simulink model "test_pkt_fifo_10_1"  (Simulink 7.0)
settings: Solver=ode45  StartTime=0.0  StopTime=2000  RelTol=1e-3
libraries: xbsIndex_r4 x102, xps_library x7, xbsReplacements_r4 x4, casper_library x3
settings Model: Creator=Jason Manley  LastModifiedBy=dsp
settings DebuggingCC: SaveWithParameterizedLinksMsg=none  SignalResolutionControl=TryResolveAllWithWarning  MultiTaskDSMMsg=warning  MultiTaskCondExecSysMsg=none  StrictBusMsg=None
settings RTWCC: IncludeERTFirstTime=on
settings GRTTargetCC: TargetFcnLib=ansi_tfl_tmw.mat

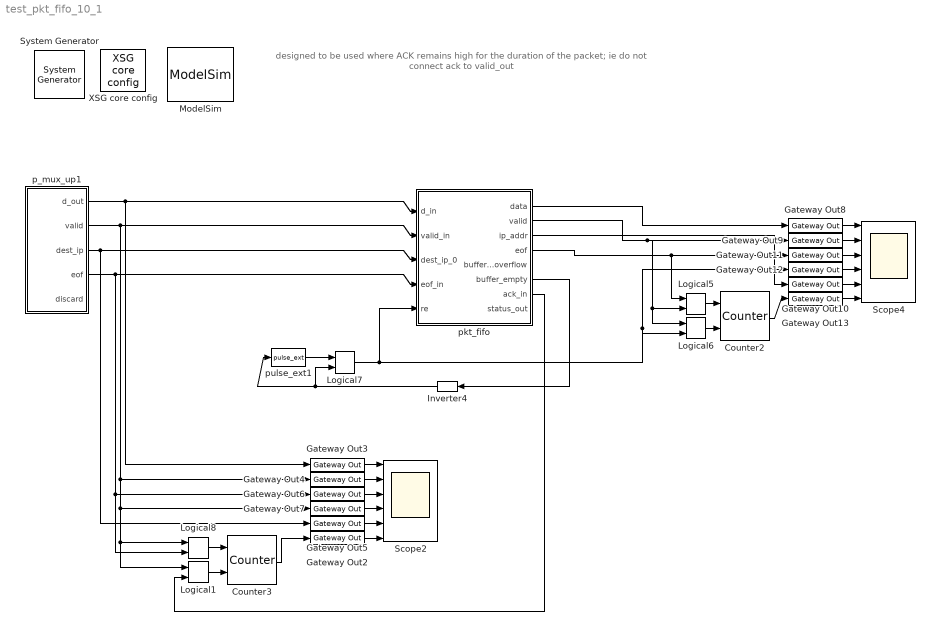
== system test_pkt_fifo_10_1 ==
  note: designed to be used where ACK remains high for the duration of the packet;
      | ie do not connect ack to valid_out
  " System Generator" : xbsIndex_r4/ System Generator  Tag=genX  SystemSampleTime=-1  xilinxfamily=Virtex2P  part=xc2vp70  speed=-7  package=ff1704  synthesis_tool=XST  clock_wrapper=Clock Enables  directory=./test_10gbe_mux_pack/sysgen  testbench=off  simulink_period=1  sysclk_period=4.878  dcm_input_clock_period=100  incr_netlist=off  trim_vbits=Everywhere in SubSystem  dbl_ovrd=According to Block Masks  core_generation=According to Block Masks  run_coregen=off  deprecated_control=off  eval_field=0  block_type=sysgen
      settings: block_version=10.1.3
  Counter2 : xbsIndex_r4/Counter  cnt_type=Free Running  cnt_to=Inf  operation=Up  start_count=0  cnt_by_val=1  arith_type=Unsigned  n_bits=8  bin_pt=0  load_pin=off  rst=on  en=on  explicit_period=off  period=1  dbl_ovrd=off  use_behavioral_HDL=off  use_rpm=on  implementation=Fabric  block_type=counter
      settings: xl_area=[0, 0, 0, 0, 0, 0, 0]
  Counter3 : xbsIndex_r4/Counter  cnt_type=Free Running  cnt_to=Inf  operation=Up  start_count=0  cnt_by_val=1  arith_type=Unsigned  n_bits=8  bin_pt=0  load_pin=off  rst=on  en=on  explicit_period=off  period=1  dbl_ovrd=off  use_behavioral_HDL=off  use_rpm=on  implementation=Fabric  block_type=counter
      settings: xl_area=[0, 0, 0, 0, 0, 0, 0]
  Gateway Out{2..13} (12 alike) : xbsIndex_r4/Gateway Out  hdl_port=on  timing_constraint=None  locs_specified=off  LOCs={}  block_type=gatewayout
      settings: infoedit="Gateway out block.  Converts Xilinx fixed point inputs into ouputs of type Simulink integer, double, or fixed point.<P><P>Hardware notes:  In hardware these blocks become top level output ports or are discarded, depending on how they are configured."  xl_area=[0, 0, 0, 0, 0, 0, 0]  block_version=10.1.3
  Inverter4 : xbsIndex_r4/Inverter  Orientation=left  en=off  latency=0  dbl_ovrd=off  block_type=inv
      settings: xl_area=[0, 0, 0, 0, 0, 0, 0]
  Logical{1,5..6,8} (4 alike) : xbsIndex_r4/Logical  logical_function=AND  inputs=2  en=off  latency=0  precision=Full  arith_type=Unsigned  n_bits=8  bin_pt=2  align_bp=on  dbl_ovrd=off  block_type=logical
      settings: xl_area=[0, 0, 0, 0, 0, 0, 0]
  Logical7 : xbsIndex_r4/Logical  logical_function=OR  inputs=2  en=off  latency=0  precision=Full  arith_type=Unsigned  n_bits=8  bin_pt=2  align_bp=on  dbl_ovrd=off  block_type=logical
      settings: xl_area=[0, 0, 0, 0, 0, 0, 0]
  ModelSim : xbsIndex_r4/ModelSim  dir=./modelsim  waveform=on  leave_open=on  skip_compile=off  use_unisim=off  custom_scripts=off  startup_timeout=40  block_type=hdlcosim
      settings: infoedit="Allow other blocks to schedule HDL co-simulation tasks.<P><P>Note that selecting \"Skip compilation\" when inappropriate can cause simulation errors and failures. Please refer to the block help for details."  block_version=10.1.3
  Scope2 : Scope  NumInputPorts=6
      settings: YMin=410.4~-1~-1~-1~0~-5  YMax=453.6~1~1~1~1~5  SaveName=ScopeData5
  Scope4 : Scope  NumInputPorts=6
      settings: YMin=410.4~-1~-1~-1~0~-5  YMax=453.6~1~1~1~1~5  SaveName=ScopeData7
  XSG core config : xps_library/XSG core config  Tag=xps:xsg  SystemSampleTime=-1  hw_sys=BEE2_usr  ibob_linux=off  clk_src=sys_clk  iBOB_clk_src=sys_clk  BEE2_ctrl_clk_src=sys_clk  BEE2_usr_clk_src=sys_clk  ROACH_clk_src=arb_clk  CORR_clk_src=sys_clk  gpio_clk_io_group=iBOB:sma  gpio_clk_bit_index=0  clk_rate=100  sample_period=1  synthesis_tool=XST  mpc_type=powerpc405
  p_mux_up1 : Subsystem
  pkt_fifo : Subsystem
      settings: AttributesFormatString=|
      | Max 1024 data words.
      | Max 32 pkts.
  pulse_ext1 : casper_library/Misc/pulse_ext  SystemSampleTime=-1  pulse_len=10
  wires:
  Gateway Out8/1 -> Scope4/1
  Gateway Out9/1 -> Scope4/2
  Gateway Out11/1 -> Scope4/3
  Gateway Out12/1 -> Scope4/4
  Gateway Out10/1 -> Scope4/5
  Gateway Out13/1 -> Scope4/6
  Gateway Out3/1 -> Scope2/1
  Gateway Out4/1 -> Scope2/2
  Gateway Out6/1 -> Scope2/3
  Gateway Out7/1 -> Scope2/4
  Gateway Out5/1 -> Scope2/5
  p_mux_up1/1(d_out) -> Gateway Out3/1, pkt_fifo/1(d_in)
  p_mux_up1/2(valid) -> Gateway Out4/1, Gateway Out7/1, Logical8/1, Logical1/1, pkt_fifo/2(valid_in)
  p_mux_up1/3(dest_ip) -> Gateway Out5/1, pkt_fifo/3(dest_ip_0)
  p_mux_up1/4(eof) -> Gateway Out6/1, Logical8/2, pkt_fifo/4(eof_in)
  pkt_fifo/1(data) -> Gateway Out8/1
  pkt_fifo/2(valid) -> Gateway Out9/1, Logical5/2, Logical6/1
  Logical5/1 -> Counter2/1
  Counter2/1 -> Gateway Out13/1
  pkt_fifo/4(eof) -> Logical5/1, Gateway Out11/1
  Logical7/1 -> Gateway Out12/1, Logical6/2, pkt_fifo/5(re)
  pkt_fifo/3(ip_addr) -> Gateway Out10/1
  Logical6/1 -> Counter2/2
  pulse_ext1/1 -> Logical7/1
  Logical8/1 -> Counter3/1
  Logical1/1 -> Counter3/2
  Gateway Out2/1 -> Scope2/6
  Counter3/1 -> Gateway Out2/1
  pkt_fifo/7(ack_in) -> Logical1/2
  pkt_fifo/6(buffer_empty) -> Inverter4/1
  Inverter4/1 -> pulse_ext1/1, Logical7/2

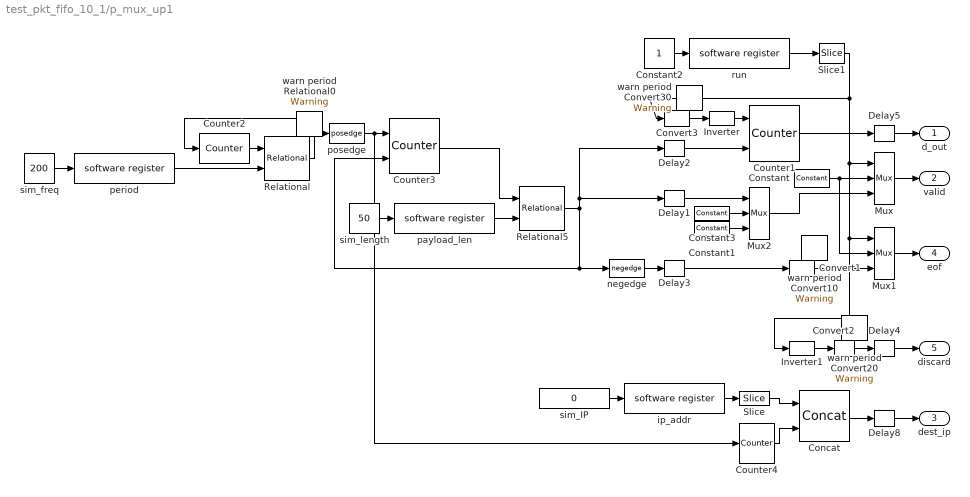
== system test_pkt_fifo_10_1/p_mux_up1 ==
  Concat : xbsIndex_r4/Concat  num_inputs=2  dbl_ovrd=off  block_type=concat
      settings: block_version=10.1.3
  Constant : xbsIndex_r4/Constant  arith_type=Boolean  const=0  n_bits=1  bin_pt=0  explicit_period=on  period=1  equ=P=C  opselect=C  inp2=PCIN>>17  opr=+  inp1=P  carry=CIN  dbl_ovrd=off  block_type=constant
  Constant1 : xbsIndex_r4/Constant  arith_type=Boolean  const=1  n_bits=1  bin_pt=0  explicit_period=off  period=1  equ=P=C  opselect=C  inp2=PCIN>>17  opr=+  inp1=P  carry=CIN  dbl_ovrd=off  block_type=constant
  Constant2 : Constant  OutDataType=sfix(16)  OutScaling=2^0
  Constant3 : xbsIndex_r4/Constant  arith_type=Boolean  const=0  n_bits=1  bin_pt=0  explicit_period=off  period=1  equ=P=C  opselect=C  inp2=PCIN>>17  opr=+  inp1=P  carry=CIN  dbl_ovrd=off  block_type=constant
  Convert1 : xbsIndex_r4/Convert  arith_type=Boolean  n_bits=8  bin_pt=6  quantization=Truncate  overflow=Wrap  latency=0  dbl_ovrd=off  pipeline=off  block_type=convert
      settings: xl_area=[0, 0, 0, 0, 0, 0, 0]  block_version=10.1.3
  Convert2 : xbsIndex_r4/Convert  arith_type=Boolean  n_bits=8  bin_pt=6  quantization=Truncate  overflow=Wrap  latency=0  dbl_ovrd=off  pipeline=off  block_type=convert
      settings: xl_area=[0, 0, 0, 0, 0, 0, 0]  block_version=10.1.3
  Convert3 : xbsIndex_r4/Convert  arith_type=Boolean  n_bits=8  bin_pt=6  quantization=Truncate  overflow=Wrap  latency=0  dbl_ovrd=off  pipeline=off  block_type=convert
      settings: xl_area=[0, 0, 0, 0, 0, 0, 0]  block_version=10.1.3
  Counter1 : xbsIndex_r4/Counter  cnt_type=Free Running  cnt_to=Inf  operation=Up  start_count=0  cnt_by_val=1  arith_type=Unsigned  n_bits=64  bin_pt=0  load_pin=off  rst=on  en=on  explicit_period=off  period=1  dbl_ovrd=off  use_behavioral_HDL=off  use_rpm=off  implementation=Fabric  block_type=counter
      settings: xl_area=[0, 0, 0, 0, 0, 0, 0]
  Counter2 : xbsIndex_r4/Counter  cnt_type=Free Running  cnt_to=Inf  operation=Up  start_count=1  cnt_by_val=1  arith_type=Unsigned  n_bits=32  bin_pt=0  load_pin=off  rst=on  en=off  explicit_period=on  period=1  dbl_ovrd=off  use_behavioral_HDL=off  use_rpm=on  implementation=Fabric  block_type=counter
      settings: xl_area=[0, 0, 0, 0, 0, 0, 0]
  Counter3 : xbsIndex_r4/Counter  cnt_type=Free Running  cnt_to=1023  operation=Up  start_count=0  cnt_by_val=1  arith_type=Unsigned  n_bits=32  bin_pt=0  load_pin=off  rst=on  en=on  explicit_period=on  period=1  dbl_ovrd=off  use_behavioral_HDL=off  use_rpm=on  implementation=Fabric  block_type=counter
      settings: xl_area=[0, 0, 0, 0, 0, 0, 0]
  Counter4 : xbsIndex_r4/Counter  cnt_type=Free Running  cnt_to=1023  operation=Up  start_count=0  cnt_by_val=1  arith_type=Unsigned  n_bits=2  bin_pt=0  load_pin=off  rst=off  en=on  explicit_period=on  period=1  dbl_ovrd=off  use_behavioral_HDL=off  use_rpm=on  implementation=Fabric  block_type=counter
      settings: xl_area=[0, 0, 0, 0, 0, 0, 0]
  Delay{1..5} (5 alike) : xbsIndex_r4/Delay  en=off  latency=1  dbl_ovrd=off  reg_retiming=on  block_type=delay
      settings: xl_area=[0, 0, 0, 0, 0, 0, 0]
  Delay8 : xbsIndex_r4/Delay  en=off  latency=2  dbl_ovrd=off  reg_retiming=on  block_type=delay
      settings: xl_area=[0, 0, 0, 0, 0, 0, 0]
  Inverter : xbsIndex_r4/Inverter  en=off  latency=0  dbl_ovrd=off  block_type=inv
      settings: xl_area=[0, 0, 0, 0, 0, 0, 0]
  Inverter1 : xbsIndex_r4/Inverter  en=off  latency=0  dbl_ovrd=off  block_type=inv
      settings: xl_area=[0, 0, 0, 0, 0, 0, 0]
  Mux : xbsIndex_r4/Mux  inputs=2  en=off  latency=1  precision=Full  arith_type="Signed  (2's comp)"  n_bits=8  bin_pt=2  quantization=Truncate  overflow=Wrap  dbl_ovrd=off  block_type=mux
      settings: xl_area=[0, 0, 0, 0, 0, 0, 0]
  Mux1 : xbsIndex_r4/Mux  inputs=2  en=off  latency=1  precision=Full  arith_type="Signed  (2's comp)"  n_bits=8  bin_pt=2  quantization=Truncate  overflow=Wrap  dbl_ovrd=off  block_type=mux
      settings: xl_area=[0, 0, 0, 0, 0, 0, 0]
  Mux2 : xbsIndex_r4/Mux  inputs=2  en=off  latency=1  precision=Full  arith_type="Signed  (2's comp)"  n_bits=8  bin_pt=2  quantization=Truncate  overflow=Wrap  dbl_ovrd=off  block_type=mux
      settings: xl_area=[0, 0, 0, 0, 0, 0, 0]
  Relational : xbsIndex_r4/Relational  mode=a>=b  en=off  latency=0  dbl_ovrd=off  block_type=relational
      settings: xl_area=[0, 0, 0, 0, 0, 0, 0]  block_version=10.1.3
  Relational5 : xbsIndex_r4/Relational  mode=a<b  en=off  latency=0  dbl_ovrd=off  block_type=relational
      settings: xl_area=[0, 0, 0, 0, 0, 0, 0]  block_version=10.1.3
  Slice : xbsIndex_r4/Slice  nbits=30  boolean_output=off  mode=Upper Bit Location + Width  bit1=0  base1=MSB of Input  bit0=0  base0=LSB of Input  dbl_ovrd=off  block_type=slice
      settings: infoedit="Extracts a given range of bits from each input sample and presents it at the output.  The output type is ordinarily unsigned with binary point at zero, but can be Boolean when the slice is one bit wide.<P><P>Hardware notes: In hardware this block costs nothing."  block_version=10.1.3
  Slice1 : xbsIndex_r4/Slice  nbits=1  boolean_output=off  mode=Lower Bit Location + Width  bit1=1  base1=MSB of Input  bit0=0  base0=LSB of Input  dbl_ovrd=off  block_type=slice
      settings: infoedit="Extracts a given range of bits from each input sample and presents it at the output.  The output type is ordinarily unsigned with binary point at zero, but can be Boolean when the slice is one bit wide.<P><P>Hardware notes: In hardware this block costs nothing."  block_version=10.1.3
  ip_addr : xps_library/software register  Tag=xps:sw_reg  SystemSampleTime=-1  io_dir=From Processor  arith_type=Unsigned  bitwidth=32  bin_pt=0  sample_period=1  gw_name=test_pkt_fifo_10_1_p_mux_up1_ip_addr_user_data_out
      link override test_pkt_buffer_10_1_p_mux_up1_ip_addr_user_data_out: arith_type=Unsigned  n_bits=32  bin_pt=0  period=1
      link override test_pkt_fifo_10_1_p_mux_up1_ip_addr_user_data_out: arith_type=Unsigned  n_bits=32  bin_pt=0  period=1
  negedge : casper_library/Misc/negedge  Tag=Rising Edge Detector  SystemSampleTime=-1
  payload_len : xps_library/software register  Tag=xps:sw_reg  SystemSampleTime=-1  io_dir=From Processor  arith_type=Unsigned  bitwidth=32  bin_pt=0  sample_period=1  gw_name=test_pkt_fifo_10_1_p_mux_up1_payload_len_user_data_out
      link override test_pkt_buffer_10_1_p_mux_up1_payload_len_user_data_out: arith_type=Unsigned  n_bits=32  bin_pt=0  period=1
      link override test_pkt_fifo_10_1_p_mux_up1_payload_len_user_data_out: arith_type=Unsigned  n_bits=32  bin_pt=0  period=1
  period : xps_library/software register  Tag=xps:sw_reg  SystemSampleTime=-1  io_dir=From Processor  arith_type=Unsigned  bitwidth=32  bin_pt=0  sample_period=1  gw_name=test_pkt_fifo_10_1_p_mux_up1_period_user_data_out
      link override test_pkt_buffer_10_1_p_mux_up1_period_user_data_out: arith_type=Unsigned  n_bits=32  bin_pt=0  period=1
      link override test_pkt_fifo_10_1_p_mux_up1_period_user_data_out: arith_type=Unsigned  n_bits=32  bin_pt=0  period=1
  posedge : casper_library/Misc/pulse_ext/posedge  Tag=Rising Edge Detector  SystemSampleTime=-1
  run : xps_library/software register  Tag=xps:sw_reg  SystemSampleTime=-1  io_dir=From Processor  arith_type=Unsigned  bitwidth=32  bin_pt=0  sample_period=1  gw_name=test_pkt_fifo_10_1_p_mux_up1_run_user_data_out
      link override test_pkt_buffer_10_1_p_mux_up1_run_user_data_out: arith_type=Unsigned  n_bits=32  bin_pt=0  period=1
      link override test_pkt_fifo_10_1_p_mux_up1_run_user_data_out: arith_type=Unsigned  n_bits=32  bin_pt=0  period=1
  sim_IP : Constant  Value=0  OutDataType=sfix(16)  OutScaling=2^0
  sim_freq : Constant  Value=200  OutDataType=sfix(16)  OutScaling=2^0
  sim_length : Constant  Value=50  OutDataType=sfix(16)  OutScaling=2^0
  warn period Convert10 : xbsReplacements_r4/Warning  SystemSampleTime=-1  period=1
  warn period Convert20 : xbsReplacements_r4/Warning  SystemSampleTime=-1  period=1
  warn period Convert30 : xbsReplacements_r4/Warning  SystemSampleTime=-1  period=1
  warn period Relational0 : xbsReplacements_r4/Warning  SystemSampleTime=-1  period=1
  d_out : Outport  OutDataType=sfix(16)  OutScaling=2^0
  valid : Outport  Port=2  OutDataType=sfix(16)  OutScaling=2^0
  dest_ip : Outport  Port=3  OutDataType=sfix(16)  OutScaling=2^0
  eof : Outport  Port=4  OutDataType=sfix(16)  OutScaling=2^0
  discard : Outport  Port=5  OutDataType=sfix(16)  OutScaling=2^0
  wires:
  Counter2/1 -> Relational/1
  Relational/1 -> posedge/1, Counter2/1
  Counter1/1 -> Delay5/1
  negedge/1 -> Delay3/1
  period/1 -> Relational/2
  sim_freq/1 -> period/1
  sim_IP/1 -> ip_addr/1
  Relational5/1 -> Counter3/2, negedge/1, Delay2/1, Delay1/1
  Counter3/1 -> Relational5/1
  posedge/1 -> Counter3/1, Counter4/1
  sim_length/1 -> payload_len/1
  payload_len/1 -> Relational5/2
  Mux/1 -> valid/1
  Constant/1 -> Mux/2, Mux1/2
  Mux1/1 -> eof/1
  Delay3/1 -> Convert1/1
  Convert1/1 -> Mux1/3
  Delay5/1 -> d_out/1
  Delay8/1 -> dest_ip/1
  run/1 -> Slice1/1
  Constant2/1 -> run/1
  Slice1/1 -> Mux/1, Mux1/1, Inverter1/1, Convert3/1
  Delay4/1 -> discard/1
  Mux2/1 -> Mux/3
  Inverter/1 -> Counter1/1
  Delay2/1 -> Counter1/2
  Convert3/1 -> Inverter/1
  Constant3/1 -> Mux2/2
  Constant1/1 -> Mux2/3
  Inverter1/1 -> Convert2/1
  Delay1/1 -> Mux2/1
  Convert2/1 -> Delay4/1
  ip_addr/1 -> Slice/1
  Counter4/1 -> Concat/2
  Slice/1 -> Concat/1
  Concat/1 -> Delay8/1

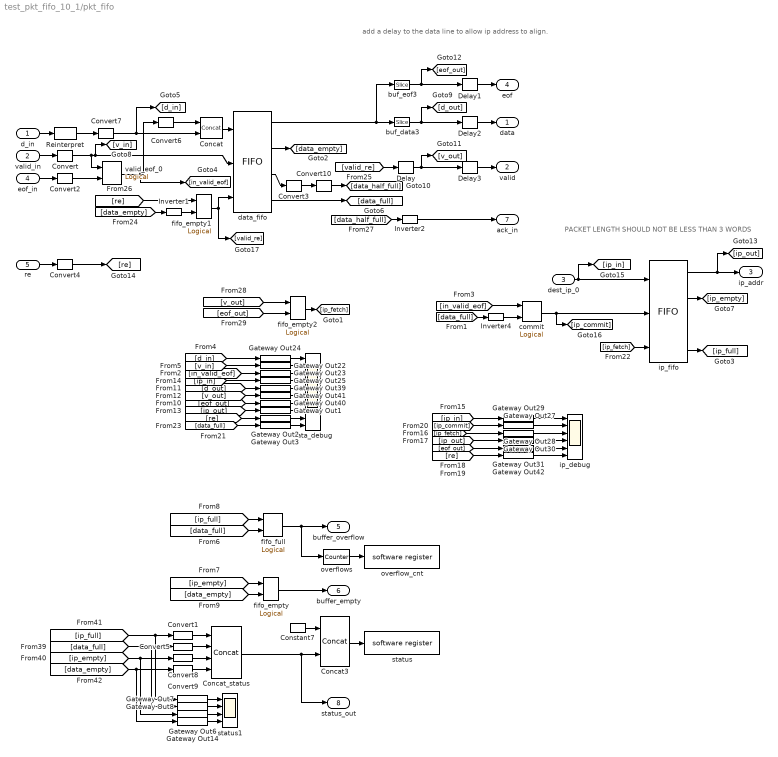
== system test_pkt_fifo_10_1/pkt_fifo ==
  note: PACKET LENGTH SHOULD NOT BE LESS THAN 3 WORDS
  note: add a delay to the data line to allow
      | ip address to align.
  d_in : Inport  OutDataType=sfix(16)  OutScaling=2^0
  valid_in : Inport  Port=2  OutDataType=sfix(16)  OutScaling=2^0
  dest_ip_0 : Inport  Port=3  OutDataType=sfix(16)  OutScaling=2^0
  eof_in : Inport  Port=4  OutDataType=sfix(16)  OutScaling=2^0
  re : Inport  Port=5  OutDataType=sfix(16)  OutScaling=2^0
  Concat : xbsIndex_r4/Concat  num_inputs=2  dbl_ovrd=off  block_type=concat
      settings: block_version=10.1.3
  Concat3 : xbsIndex_r4/Concat  num_inputs=2  dbl_ovrd=off  block_type=concat
      settings: block_version=10.1.3
  Concat_status : xbsIndex_r4/Concat  num_inputs=4  dbl_ovrd=off  block_type=concat
      settings: block_version=10.1.3
  Constant7 : xbsIndex_r4/Constant  arith_type=Unsigned  const=0  n_bits=32-9  bin_pt=0  explicit_period=on  period=1  equ=P=C  opselect=C  inp2=PCIN>>17  opr=+  inp1=P  carry=CIN  dbl_ovrd=off  block_type=constant
  Convert : xbsIndex_r4/Convert  arith_type=Boolean  n_bits=8  bin_pt=6  quantization=Truncate  overflow=Wrap  latency=0  dbl_ovrd=off  pipeline=off  block_type=convert
      settings: xl_area=[0, 0, 0, 0, 0, 0, 0]  block_version=10.1.3
  Convert{1,3,5..6,8..9} (6 alike) : xbsIndex_r4/Convert  arith_type=Unsigned  n_bits=1  bin_pt=0  quantization=Truncate  overflow=Wrap  latency=0  dbl_ovrd=off  pipeline=off  block_type=convert
      settings: xl_area=[0, 0, 0, 0, 0, 0, 0]  block_version=10.1.3
  Convert10 : xbsIndex_r4/Convert  arith_type=Boolean  n_bits=1  bin_pt=0  quantization=Truncate  overflow=Wrap  latency=0  dbl_ovrd=off  pipeline=off  block_type=convert
      settings: xl_area=[0, 0, 0, 0, 0, 0, 0]  block_version=10.1.3
  Convert2 : xbsIndex_r4/Convert  arith_type=Boolean  n_bits=8  bin_pt=6  quantization=Truncate  overflow=Wrap  latency=0  dbl_ovrd=off  pipeline=off  block_type=convert
      settings: xl_area=[0, 0, 0, 0, 0, 0, 0]  block_version=10.1.3
  Convert4 : xbsIndex_r4/Convert  arith_type=Boolean  n_bits=8  bin_pt=6  quantization=Truncate  overflow=Wrap  latency=0  dbl_ovrd=off  pipeline=off  block_type=convert
      settings: xl_area=[0, 0, 0, 0, 0, 0, 0]  block_version=10.1.3
  Convert7 : xbsIndex_r4/Convert  arith_type=Unsigned  n_bits=64  bin_pt=0  quantization=Truncate  overflow=Wrap  latency=0  dbl_ovrd=off  pipeline=off  block_type=convert
      settings: xl_area=[0, 0, 0, 0, 0, 0, 0]  block_version=10.1.3
  Delay{,1..3} (4 alike) : xbsIndex_r4/Delay  en=off  latency=1  dbl_ovrd=off  reg_retiming=off  block_type=delay
  Gateway Out{1..3,6..8,14,22..25,27..31,39..42} (20 alike) : xbsIndex_r4/Gateway Out  hdl_port=on  timing_constraint=None  locs_specified=off  LOCs={}  block_type=gatewayout
      settings: infoedit="Gateway out block.  Converts Xilinx fixed point inputs into ouputs of type Simulink integer, double, or fixed point.<P><P>Hardware notes:  In hardware these blocks become top level output ports or are discarded, depending on how they are configured."  xl_area=[0, 0, 0, 0, 0, 0, 0]  block_version=10.1.3
  Inverter1 : xbsIndex_r4/Inverter  en=off  latency=0  dbl_ovrd=off  block_type=inv
      settings: xl_area=[0, 0, 0, 0, 0, 0, 0]
  Inverter2 : xbsIndex_r4/Inverter  en=off  latency=0  dbl_ovrd=off  block_type=inv
      settings: xl_area=[0, 0, 0, 0, 0, 0, 0]
  Inverter4 : xbsIndex_r4/Inverter  en=off  latency=0  dbl_ovrd=off  block_type=inv
      settings: xl_area=[0, 0, 0, 0, 0, 0, 0]
  Reinterpret : xbsIndex_r4/Reinterpret  force_arith_type=on  arith_type=Unsigned  force_bin_pt=on  bin_pt=0  block_type=reinterpret
      settings: infoedit="Changes signal type without altering the binary representation.   You can changed the signal between signed and unsigned, and relocate the binary point.<P><P>Hardware notes: In hardware this block costs nothing.<P><P>Example:  Suppose the input is 6 bits wide, signed, with 2 fractional bits, and the output is forced to unsigned with 0 fractional bits.  Then an input of -2.0 (1110.00 in binary 2's complement) becomes an output of 56 (111000 in binary)."  block_version=10.1.3
  buf_data3 : xbsIndex_r4/Slice  nbits=64  boolean_output=off  mode=Lower Bit Location + Width  bit1=33  base1=LSB of Input  bit0=0  base0=LSB of Input  dbl_ovrd=off  block_type=slice
      settings: infoedit="Extracts a given range of bits from each input sample and presents it at the output.  The output type is ordinarily unsigned with binary point at zero, but can be Boolean when the slice is one bit wide.<P><P>Hardware notes: In hardware this block costs nothing."  block_version=10.1.3
  buf_eof3 : xbsIndex_r4/Slice  nbits=1  boolean_output=on  mode=Upper Bit Location + Width  bit1=64  base1=LSB of Input  bit0=0  base0=LSB of Input  dbl_ovrd=off  block_type=slice
      settings: infoedit="Extracts a given range of bits from each input sample and presents it at the output.  The output type is ordinarily unsigned with binary point at zero, but can be Boolean when the slice is one bit wide.<P><P>Hardware notes: In hardware this block costs nothing."  block_version=10.1.3
  commit : xbsIndex_r4/Logical  logical_function=AND  inputs=2  en=off  latency=0  precision=Full  arith_type=Unsigned  n_bits=8  bin_pt=2  align_bp=on  dbl_ovrd=off  block_type=logical
      settings: xl_area=[0, 0, 0, 0, 0, 0, 0]
  data_debug : Scope  NumInputPorts=10
      settings: YMin=12000~0~9500~0~15500~0~0~-5~-5~-5  YMax=13300~1~10500~1~17250~1~1~5~5~5  SaveName=ScopeData8
  data_fifo : xbsIndex_r4/FIFO  depth=128  percent_nbits=1  rst=off  en=off  use_dcount=off  use_almost_empty=off  almost_empty_thresh=2  use_almost_full=off  almost_full_thresh=14  dbl_ovrd=off  mem_type=Block RAM  block_type=fifo
      settings: block_version=10.1.3
  fifo_empty : xbsIndex_r4/Logical  logical_function=AND  inputs=2  en=off  latency=0  precision=Full  arith_type=Unsigned  n_bits=8  bin_pt=2  align_bp=on  dbl_ovrd=off  block_type=logical
      settings: xl_area=[0, 0, 0, 0, 0, 0, 0]
  fifo_empty1 : xbsIndex_r4/Logical  logical_function=AND  inputs=2  en=off  latency=0  precision=Full  arith_type=Unsigned  n_bits=8  bin_pt=2  align_bp=on  dbl_ovrd=off  block_type=logical
      settings: xl_area=[0, 0, 0, 0, 0, 0, 0]
  fifo_empty2 : xbsIndex_r4/Logical  logical_function=AND  inputs=2  en=off  latency=0  precision=Full  arith_type=Unsigned  n_bits=8  bin_pt=2  align_bp=on  dbl_ovrd=off  block_type=logical
      settings: xl_area=[0, 0, 0, 0, 0, 0, 0]
  fifo_full : xbsIndex_r4/Logical  logical_function=OR  inputs=2  en=off  latency=0  precision=Full  arith_type=Unsigned  n_bits=8  bin_pt=2  align_bp=on  dbl_ovrd=off  block_type=logical
      settings: xl_area=[0, 0, 0, 0, 0, 0, 0]
  ip_debug : Scope  NumInputPorts=6
      settings: YMin=100~0~0~100~0~-5  YMax=103~1~1~103~1~5  SaveName=ScopeData9
  ip_fifo : xbsIndex_r4/FIFO  depth=64  percent_nbits=2  rst=off  en=off  use_dcount=off  use_almost_empty=off  almost_empty_thresh=2  use_almost_full=off  almost_full_thresh=14  dbl_ovrd=off  mem_type=Block RAM  block_type=fifo
      settings: block_version=10.1.3
  overflow_cnt : xps_library/software register  Tag=xps:sw_reg  SystemSampleTime=-1  io_dir=To Processor  arith_type=Unsigned  bitwidth=32  bin_pt=0  sample_period=1  gw_name=test_pkt_fifo_10_1_pkt_buffer_new_overflow_cnt_user_data_in
      link override convert: arith_type=Unsigned  n_bits=32  bin_pt=0
  overflows : xbsIndex_r4/Counter  cnt_type=Free Running  cnt_to=Inf  operation=Up  start_count=0  cnt_by_val=1  arith_type=Unsigned  n_bits=32  bin_pt=0  load_pin=off  rst=off  en=on  explicit_period=off  period=1  dbl_ovrd=off  use_behavioral_HDL=off  use_rpm=on  implementation=Fabric  block_type=counter
      settings: xl_area=[0, 0, 0, 0, 0, 0, 0]
  status : xps_library/software register  Tag=xps:sw_reg  SystemSampleTime=-1  io_dir=To Processor  arith_type=Unsigned  bitwidth=32  bin_pt=0  sample_period=1  gw_name=test_pkt_fifo_10_1_pkt_buffer_new_status_user_data_in
      link override convert: arith_type=Unsigned  n_bits=32  bin_pt=0
  status1 : Scope  NumInputPorts=4
      settings: YMin=-1~-1~-1~-1  YMax=1~1~1~1  SaveName=ScopeData6
  valid_eof_0 : xbsIndex_r4/Logical  logical_function=AND  inputs=2  en=off  latency=0  precision=Full  arith_type=Unsigned  n_bits=8  bin_pt=2  align_bp=on  dbl_ovrd=off  block_type=logical
      settings: xl_area=[0, 0, 0, 0, 0, 0, 0]
  data : Outport  OutDataType=sfix(16)  OutScaling=2^0
  valid : Outport  Port=2  OutDataType=sfix(16)  OutScaling=2^0
  ip_addr : Outport  Port=3  OutDataType=sfix(16)  OutScaling=2^0
  eof : Outport  Port=4  OutDataType=sfix(16)  OutScaling=2^0
  buffer_overflow : Outport  Port=5  OutDataType=sfix(16)  OutScaling=2^0
  buffer_empty : Outport  Port=6  OutDataType=sfix(16)  OutScaling=2^0
  ack_in : Outport  Port=7  OutDataType=sfix(16)  OutScaling=2^0
  status_out : Outport  Port=8  OutDataType=sfix(16)  OutScaling=2^0
  wires:
  [data_full] -> Gateway Out3/1
  Gateway Out3/1 -> data_debug/10
  Convert4/1 -> [re]
  Convert2/1 -> valid_eof_0/2
  Convert/1 -> [v_in], data_fifo/2, valid_eof_0/1
  Reinterpret/1 -> Convert7/1
  [ip_fetch] -> ip_fifo/3
  [re] -> Gateway Out2/1
  Gateway Out2/1 -> data_debug/9
  [ip_fetch] -> Gateway Out28/1
  [data_full] -> Inverter4/1
  [ip_commit] -> Gateway Out27/1
  [re] -> Gateway Out42/1
  re/1 -> Convert4/1
  [eof_out] -> Gateway Out31/1
  [ip_out] -> Gateway Out30/1
  [ip_in] -> Gateway Out29/1
  [in_valid_eof] -> Gateway Out23/1
  [v_in] -> Gateway Out22/1
  [d_in] -> Gateway Out24/1
  [ip_in] -> Gateway Out25/1
  [d_out] -> Gateway Out39/1
  [v_out] -> Gateway Out41/1
  [eof_out] -> Gateway Out40/1
  [ip_out] -> Gateway Out1/1
  Gateway Out1/1 -> data_debug/8
  Convert9/1 -> Concat_status/4
  Convert8/1 -> Concat_status/3
  Convert5/1 -> Concat_status/2
  Convert1/1 -> Concat_status/1
  Gateway Out14/1 -> status1/4
  Gateway Out6/1 -> status1/3
  Gateway Out8/1 -> status1/2
  Gateway Out7/1 -> status1/1
  [in_valid_eof] -> commit/1
  buf_eof3/1 -> Delay1/1, [eof_out]
  buf_data3/1 -> [d_out], Delay2/1
  data_fifo/2 -> [data_empty]
  Gateway Out42/1 -> ip_debug/6
  Gateway Out40/1 -> data_debug/7
  Gateway Out41/1 -> data_debug/6
  Gateway Out39/1 -> data_debug/5
  Gateway Out31/1 -> ip_debug/5
  Gateway Out30/1 -> ip_debug/4
  Gateway Out28/1 -> ip_debug/3
  Gateway Out27/1 -> ip_debug/2
  Gateway Out29/1 -> ip_debug/1
  Gateway Out25/1 -> data_debug/4
  Gateway Out23/1 -> data_debug/3
  Gateway Out22/1 -> data_debug/2
  Gateway Out24/1 -> data_debug/1
  overflows/1 -> overflow_cnt/1
  ip_fifo/1 -> [ip_out], ip_addr/1
  data_fifo/1 -> buf_data3/1, buf_eof3/1
  valid_eof_0/1 -> [in_valid_eof], Convert6/1
  Inverter4/1 -> commit/2
  ip_fifo/2 -> [ip_empty]
  eof_in/1 -> Convert2/1
  dest_ip_0/1 -> [ip_in], ip_fifo/1
  valid_in/1 -> Convert/1
  d_in/1 -> Reinterpret/1
  commit/1 -> [ip_commit], ip_fifo/2
  ip_fifo/4 -> [ip_full]
  data_fifo/4 -> [data_full]
  Concat/1 -> data_fifo/1
  Constant7/1 -> Concat3/1
  Concat3/1 -> status/1
  Concat_status/1 -> status_out/1, Concat3/2
  [data_empty] -> Gateway Out14/1, Convert9/1
  [ip_empty] -> Gateway Out6/1, Convert8/1
  [data_full] -> Convert5/1, Gateway Out8/1
  [ip_full] -> Gateway Out7/1, Convert1/1
  [data_full] -> fifo_full/2
  [ip_full] -> fifo_full/1
  [data_empty] -> fifo_empty/2
  [ip_empty] -> fifo_empty/1
  fifo_empty/1 -> buffer_empty/1
  fifo_full/1 -> overflows/1, buffer_overflow/1
  [valid_re] -> Delay/1
  [data_empty] -> Inverter1/1
  Inverter1/1 -> fifo_empty1/2
  Delay/1 -> [v_out], Delay3/1
  [data_half_full] -> Inverter2/1
  Inverter2/1 -> ack_in/1
  data_fifo/3 -> Convert3/1
  Convert3/1 -> Convert10/1
  Convert6/1 -> Concat/1
  Convert7/1 -> [d_in], Concat/2
  Convert10/1 -> [data_half_full]
  Delay1/1 -> eof/1
  Delay2/1 -> data/1
  Delay3/1 -> valid/1
  fifo_empty2/1 -> [ip_fetch]
  [v_out] -> fifo_empty2/1
  [eof_out] -> fifo_empty2/2
  [re] -> fifo_empty1/1
  fifo_empty1/1 -> data_fifo/3, [valid_re]
